simulink model "example_F3"  (R2016b)
settings: Solver=VariableStepAuto  StartTime=0.0  StopTime=10.0  RelTol=1e-3
PreLoadFcn:
  | t = [0.0 3.0 7.0 10.0]';
  | u = [0.0 0.5 1.0 0.0]';
settings Model: Creator=training-ah  LastModifiedBy=training-ah
settings DataIOCC: LoadExternalInput=on  SaveFormat=Array

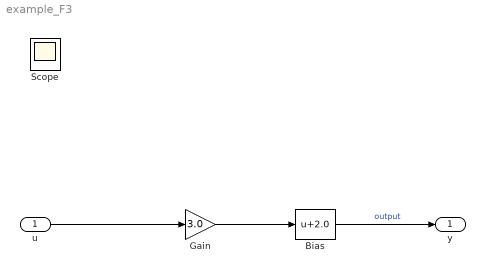
== system example_F3 ==
  "u " : Inport
  Bias : Bias  Bias=2.0
  Gain : Gain  Gain=3.0
  "y " : Outport
  Scope : Scope
  wires:
  Gain/1 -> Bias/1
  "u "/1 -> Gain/1
  Bias/1 -> "y "/1  "output"
